simulink model "LiniowyRowStanu"  (R2015a)
settings: Solver=ode45  StartTime=0.0  StopTime=200  MaxStep=0.1  RelTol=1e-3
values from neighbouring files (symbols this model uses):
  A1 = 3500    [ZbiorniczkiDokladne.m]
  A2 = 2000    [ZbiorniczkiDokladne.m]
  df1 = 200    [ZbiorniczkiDokladne.m]
  df2 = 0    [ZbiorniczkiDokladne.m]
  f1 = wektorf1(i)    [ZbiorniczkiDokladne.m]
  f2 = 0    [ZbiorniczkiDokladne.m]
  h1 = ((f1.^2)/((Aw1.^2)*2*g))+((f1+f2).^2)/((Aw2.^2)*2*g)    [ZbiorniczkiDokladne.m]
  h2 = ((f1+f2).^2)/((Aw2.^2)*2*g)    [ZbiorniczkiDokladne.m]
  t1 = 40    [ZbiorniczkiDokladne.m]
  t2 = 40    [ZbiorniczkiDokladne.m]
undefined symbols (not defined in the file or in its folder): a1, a2
settings Model: Creator=apuch  LastModifiedBy=apuch

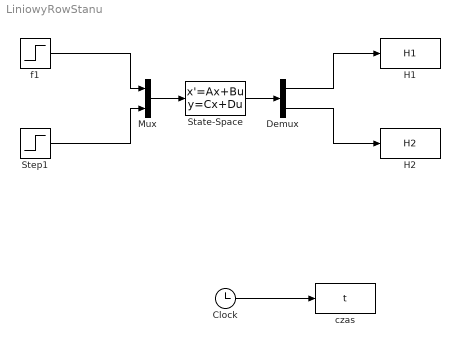
== system LiniowyRowStanu ==
  Clock : Clock
  Demux : Demux  Outputs=2
  H1 : ToWorkspace  VariableName=H1  SampleTime=-1
  H2 : ToWorkspace  VariableName=H2  SampleTime=-1
  Mux : Mux  Inputs=2
  State-Space : StateSpace  A=[-a1/A1, a1/A1; a1/A2, (-a1-a2)/A2]  B=[1/A1, 0; 0, 1/A2]  C=[1, 0; 0, 1]  D=[0, 0; 0, 0]  X0=[h1 h2]
  Step1 : Step  Time=t2  Before=f2  After=f2+df2  SampleTime=0
  czas : ToWorkspace  VariableName=t  SampleTime=-1
  f1 : Step  Time=t1  Before=f1  After=f1+df1  SampleTime=0
  wires:
  f1/1 -> Mux/1
  Step1/1 -> Mux/2
  Mux/1 -> State-Space/1
  State-Space/1 -> Demux/1
  Demux/1 -> H1/1
  Demux/2 -> H2/1
  Clock/1 -> czas/1
